simulink model "Model"  (R2020b)
settings: Solver=VariableStepAuto  StartTime=0.0  StopTime=20.0  MaxStep=0.1  RelTol=1e-3
settings Model: Creator=user  LastModifiedBy=user
settings DataIOCC: ExternalInput=[t, flor]  LoadExternalInput=on

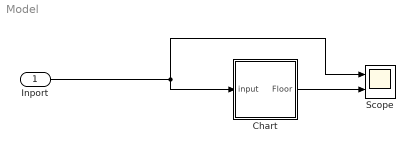
== system Model ==
  Inport : Inport  OutDataTypeStr=double  Interpolate=off
  Chart : Stateflow chart  TreatAsAtomicUnit=on
  Scope : Scope  NumInputPorts=2
  wires:
  Inport/1 -> Chart/1(input), Scope/1
  Chart/1(Floor) -> Scope/2

== stateflow chart Model/Chart ==
  state working [parallel]
    settings: executionOrder=1
    state LiftLocation
      (history)
      state Floor5
        entry:
        Floor = 5;
        opendoor = goto - Floor +1
      state Floor4
        entry:
        Floor = 4;
        opendoor = goto - Floor +1
      state Floor3
        entry:
        Floor = 3;
        opendoor = goto - Floor +1
      state Floor2
        entry:
        Floor = 2;
        opendoor = goto - Floor +1
      state Floor1
        entry:
        Floor = 1;
        opendoor = goto - Floor +1
        during:
        wait = 1+1;
      (default) -> Floor5
      Floor5 -> Floor5 [order 2] : [goto == 0]
      Floor5 -> Floor4 [order 1] : [goto<Floor]{doorOpened = 0}
      Floor4 -> Floor5 [order 2] : [goto>Floor]{doorOpened = 0}
      Floor4 -> Floor4 [order 3] : [goto == 0]
      Floor4 -> Floor3 [order 1] : [goto<Floor]{doorOpened = 0}
      Floor3 -> Floor4 [order 2] : [goto>Floor]{doorOpened = 0}
      Floor3 -> Floor3 [order 3] : [goto == 0]
      Floor3 -> Floor2 [order 1] : [goto<Floor]{doorOpened = 0}
      Floor2 -> Floor3 [order 2] : [goto>Floor]{doorOpened = 0}
      Floor2 -> Floor2 [order 3] : [goto == 0]
      Floor2 -> Floor1 [order 1] : [goto<Floor]{doorOpened = 0}
      Floor1 -> Floor2 [order 1] : [goto>Floor]{doorOpened = 0}
      Floor1 -> Floor1 [order 2] : [goto == 0]
    state LiftDoor
      state OpenDoor
        exit:
        floorReached = 1;
      state CloseDoor
        %goto = queue(1);
      (default) -> OpenDoor
      OpenDoor -> (junction 108)
      (junction 108) -> CloseDoor : after(2,sec)
    (default) -> LiftLocation
    LiftLocation -> (junction 52) : [opendoor == 1]
    (junction 52) -> LiftDoor : [doorOpened == 0]
    CloseDoor -> LiftLocation : after(1,sec){doorOpened = 1}
  state FloorQueue [parallel]
    settings: executionOrder=2
    state InitializeQueue
      en:
      n = 0;
      temp = input;
    state Checker
      en:
      checkVals(input,queue(i));
      i = i+1;
    state RemoveFirst
      entry:
      queue(i) = queue(i+1);
      i = i+1;
      floorReached = 0;
    state AddQueue
      en:
      n=n+1;
      queue(n) = temp;
      goto = queue(1);
      addVal =0;
    state IDLE
      en:
      i = 1
      addVal = 1;
      temp = input;
    (default) -> InitializeQueue
    Checker -> Checker [order 2] : [queue(i) ~=0]
    InitializeQueue -> (junction 106) : [input>0]
    Checker -> (junction 110) [order 1] : [addVal == 1]
    Checker -> IDLE [order 3]
    IDLE -> Checker [order 1] : [temp~=input]
    (junction 106) -> AddQueue : {temp = input}
    RemoveFirst -> RemoveFirst [order 1] : [queue(i)~=0]
    (junction 110) -> AddQueue : {temp = input}
    IDLE -> RemoveFirst [order 2] : [floorReached==1]
    RemoveFirst -> (junction 103) [order 2] : {n = n-1}
    AddQueue -> IDLE
    (junction 103) -> IDLE : {goto = queue(1)}
  state checkVals(data1,data2) [function]
    (default) -> (junction 86)
    (junction 86) -> (junction 87) [order 1] : [data1 == data2]
    (junction 86) -> (junction 88) [order 2]
    (junction 87) -> (junction 89) : {addVal = 0;}
    (junction 89) -> (junction 88)
    (junction 88) -> (junction 90)
  data: data1 function_input; data2 function_input; opendoor local; Floor output; doorOpened local; queue local =[0 0 0 0 0 0 0 0 0 0]; n local; temp local =0; addVal local =0; i local =1; floorReached local =0; wait local; goto local =1; input input
